simulink model "demostration"  (R2015b)
settings: Solver=ode45  SolverMode=SingleTasking  StartTime=0  StopTime=45.77  RelTol=1e-3
settings Model: Creator=wangze  LastModifiedBy=megan
settings DataIOCC: Decimation=2  LimitDataPoints=off  SaveFormat=Array
settings OptimizationCC: BlockReduction=off  BooleanDataType=off
settings DebuggingCC: SaveWithParameterizedLinksMsg=none  UnderspecifiedInitializationDetection=Classic  MergeDetectMultiDrivingBlocksExec=none  SignalResolutionControl=TryResolveAllWithWarning
settings HardwareCC: ProdBitPerLong=64  ProdHWDeviceType=Intel->x86-64 (Linux 64)  TargetUnknown=on
settings ModelReferenceCC: UpdateModelReferenceTargets=Force
settings GRTTargetCC: GeneratePreprocessorConditionals=Disable all
settings ConfigComp: CovModelRefEnable=Off  CovSFcnEnable=off

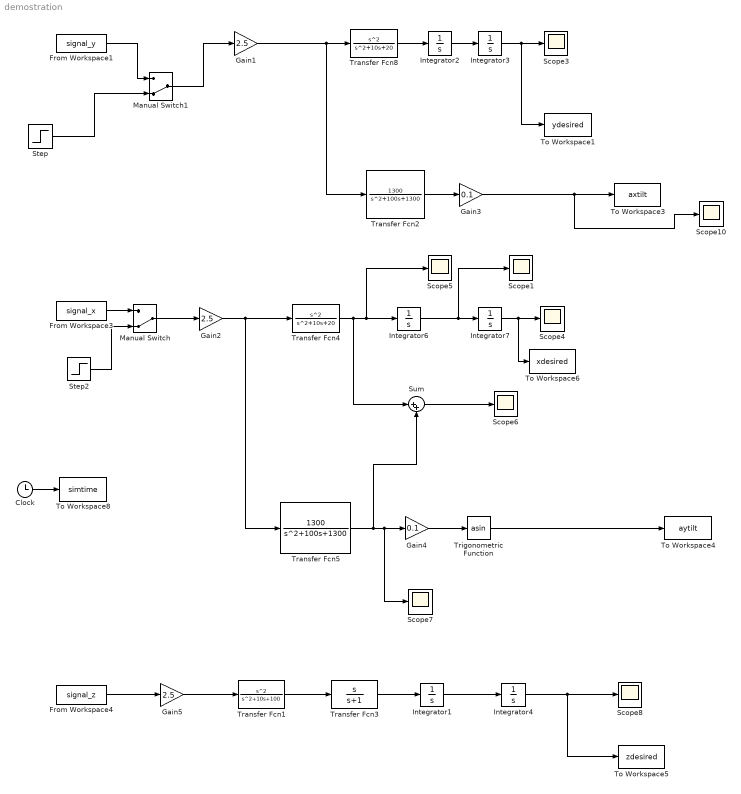
== system demostration ==
  Clock : Clock
  From Workspace1 : FromWorkspace  VariableName=signal_y
  From Workspace3 : FromWorkspace  VariableName=signal_x
  From Workspace4 : FromWorkspace  VariableName=signal_z
  Gain1 : Gain  Gain=2.5  SampleTime=0.05
  Gain2 : Gain  Gain=2.5  SampleTime=0.05
  Gain3 : Gain  Gain=0.1  SampleTime=0.05
  Gain4 : Gain  Gain=0.1  SampleTime=0.05
  Gain5 : Gain  Gain=2.5  SampleTime=0.05
  Integrator{1..4,6..7} (6 alike) : Integrator
  Manual Switch : ManualSwitch  CurrentSetting=0
  Manual Switch1 : ManualSwitch  CurrentSetting=0
  Scope{1,3..8,10} (8 alike) : Scope
  Step : Step  SampleTime=0
  Step2 : Step  Time=0  SampleTime=0
  Sum : Sum  Inputs=|++
  To Workspace1 : ToWorkspace  VariableName=ydesired  SampleTime=0.01
      settings: Decimation=2  Save2DSignal=2-D array (concatenate along first dimension)
  To Workspace3 : ToWorkspace  VariableName=axtilt  SampleTime=0.01
      settings: Decimation=2  Save2DSignal=2-D array (concatenate along first dimension)
  To Workspace4 : ToWorkspace  VariableName=aytilt  SampleTime=0.01
      settings: Decimation=2  Save2DSignal=2-D array (concatenate along first dimension)
  To Workspace5 : ToWorkspace  VariableName=zdesired  SampleTime=0.01
      settings: Decimation=2
  To Workspace6 : ToWorkspace  VariableName=xdesired  SampleTime=0.01
      settings: Decimation=2  Save2DSignal=2-D array (concatenate along first dimension)
  To Workspace8 : ToWorkspace  VariableName=simtime  SampleTime=-1
      settings: Decimation=2  Save2DSignal=2-D array (concatenate along first dimension)
  Transfer Fcn1 : TransferFcn  Numerator=[1 0 0]  Denominator=[1 10 100]
  Transfer Fcn2 : TransferFcn  Numerator=[1300]  Denominator=[1 100 1300]
  Transfer Fcn3 : TransferFcn  Numerator=[1 0]  Denominator=[1 1]
  Transfer Fcn4 : TransferFcn  Numerator=[1 0 0]  Denominator=[1 10 20]
  Transfer Fcn5 : TransferFcn  Numerator=[1300]  Denominator=[1 100 1300]
  Transfer Fcn8 : TransferFcn  Numerator=[1 0 0]  Denominator=[1 10 20]
  Trigonometric Function : Trigonometry  Operator=asin
  wires:
  Integrator2/1 -> Integrator3/1
  Integrator3/1 -> To Workspace1/1, Scope3/1
  Integrator6/1 -> Scope1/1, Integrator7/1
  Transfer Fcn4/1 -> Sum/1, Scope5/1, Integrator6/1
  Integrator7/1 -> To Workspace6/1, Scope4/1
  Gain1/1 -> Transfer Fcn2/1, Transfer Fcn8/1
  Gain4/1 -> Trigonometric Function/1
  Transfer Fcn5/1 -> Sum/2, Scope7/1, Gain4/1
  Gain2/1 -> Transfer Fcn5/1, Transfer Fcn4/1
  Manual Switch/1 -> Gain2/1
  From Workspace1/1 -> Manual Switch1/1
  Transfer Fcn8/1 -> Integrator2/1
  From Workspace4/1 -> Gain5/1
  Gain5/1 -> Transfer Fcn1/1
  Transfer Fcn1/1 -> Transfer Fcn3/1
  Transfer Fcn3/1 -> Integrator1/1
  Integrator1/1 -> Integrator4/1
  Integrator4/1 -> To Workspace5/1, Scope8/1
  Step2/1 -> Manual Switch/2
  From Workspace3/1 -> Manual Switch/1
  Sum/1 -> Scope6/1
  Transfer Fcn2/1 -> Gain3/1
  Trigonometric Function/1 -> To Workspace4/1
  Clock/1 -> To Workspace8/1
  Gain3/1 -> Scope10/1, To Workspace3/1
  Step/1 -> Manual Switch1/2
  Manual Switch1/1 -> Gain1/1
